simulink model "DSB-SC&FC"  (R2023b)
settings: Solver=VariableStepAuto  StartTime=0.0  StopTime=10.0  RelTol=1e-3
settings Model: Creator=maruv  LastModifiedBy=maruv

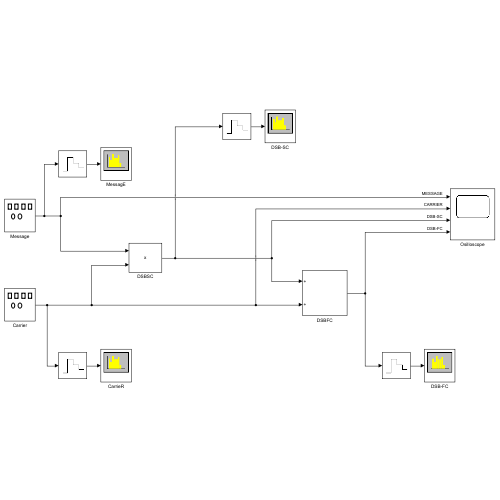
[thumbnail: Simulink's stored preview of the top-level diagram]
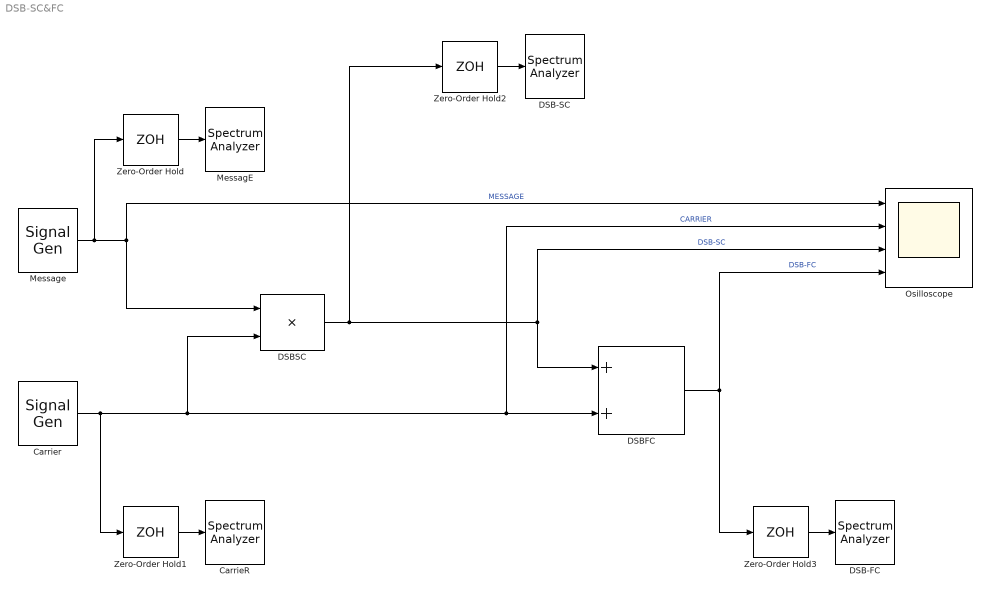
== system DSB-SC&FC ==
  CarrieR : SpectrumAnalyzer  WindowPosition=[2.000000,434.000000,766.000000,401.000000,]  Visible=on  ScopeFrameLocation=window  Span=30000  StartFrequency=-15000  StopFrequency=15000  YLimits=[-216.83306587,50.66087281]
  Carrier : SignalGenerator  Frequency=2000
  DSB-FC : SpectrumAnalyzer  WindowPosition=[770.000000,2.000000,766.000000,401.000000,]  Visible=on  ScopeFrameLocation=window  YLimits=[-216.83184174,50.66073679]
  DSB-SC : SpectrumAnalyzer  WindowPosition=[2.000000,2.000000,766.000000,401.000000,]  Visible=on  ScopeFrameLocation=window  Span=30000  StartFrequency=-15000  StopFrequency=15000  YLimits=[-256.04566642,48.40374075]
  DSBFC : Sum
  DSBSC : Product
  MessagE : SpectrumAnalyzer  WindowPosition=[770.000000,434.000000,766.000000,401.000000,]  Visible=on  ScopeFrameLocation=window  Span=4000  StartFrequency=-2000  StopFrequency=2000  YLimits=[-89.39066593,36.48778637]
  Message : SignalGenerator  Frequency=200
  Osilloscope : Scope  NumInputPorts=4
  Zero-Order Hold : ZeroOrderHold  SampleTime=1/4000
  Zero-Order Hold1 : ZeroOrderHold  SampleTime=1/30000
  Zero-Order Hold2 : ZeroOrderHold  SampleTime=1/30000
  Zero-Order Hold3 : ZeroOrderHold  SampleTime=1/30000
  wires:
  Zero-Order Hold/1 -> MessagE/1
  Message/1 -> DSBSC/1, Osilloscope/1, Zero-Order Hold/1  "MESSAGE"
  Zero-Order Hold1/1 -> CarrieR/1
  Carrier/1 -> Zero-Order Hold1/1, DSBFC/2, Osilloscope/2, DSBSC/2  "CARRIER"
  DSBSC/1 -> Zero-Order Hold2/1, Osilloscope/3, DSBFC/1  "DSB-SC"
  Zero-Order Hold2/1 -> DSB-SC/1
  Zero-Order Hold3/1 -> DSB-FC/1
  DSBFC/1 -> Zero-Order Hold3/1, Osilloscope/4  "DSB-FC"
